simulink model "bb"  (R2014a)
settings: Solver=ode45  StartTime=0.0  StopTime=200  RelTol=1e-3
settings Model: Creator=York  LastModifiedBy=York

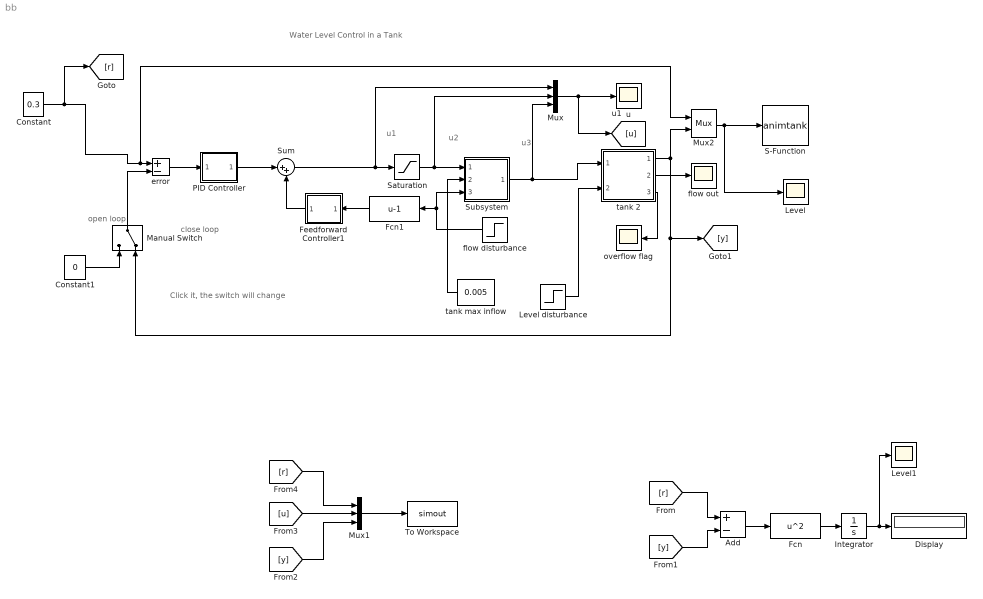
== system bb ==
  note: Water Level Control in a Tank
  note: open loop
  note: close loop
  note: Click it, the switch will change
  note: u1
  note: u2
  note: u3
  Add : Sum  Inputs=+-
  Constant : Constant  Value=0.3
  Constant1 : Constant  Value=0
  Display : Display
  Fcn : Fcn  Expr=u^2
  Fcn1 : Fcn  Expr=u-1
  Feedforward Controller1 : Subsystem  mask(feedforward Controller){K=0.002, T1=10, T2=2, t=8}
      mask prompts: K "Kffl:"; T1 "Tlead:"; T2 "Tlag:"; t "tff:"
      mask Display: disp('Gff(s)')
  Integrator : Integrator
  Level : Scope
      settings: TickLabels=on  TimeRange=200  YMin=-2.000000  YMax=2.000000  SaveName=ScopeData3
  Level disturbance : Step  Time=100  Before=1  SampleTime=0
  Level1 : Scope
      settings: TickLabels=on  TimeRange=200  YMin=-0.03  YMax=0  SaveName=ScopeData2
  Manual Switch : ManualSwitch  CurrentSetting=0
  Mux : Mux  Inputs=3
  Mux1 : Mux  Inputs=3
  Mux2 : Mux  Inputs=2
  PID Controller : Subsystem  mask(PID Controller){P=100, I=5, D=10}
      mask prompts: P "Proportional:"; I "Integral"; D "Derivative:"
      mask help:
      | Enter expressions for proportional, integral, and derivative terms.
      | P+I/s+Ds
      mask Help: This block implements a PID controller where parameters are entered for the Proportional, Integral and Derivative terms. Unmask this block to see how it works. The derivative term is implemented using a true derivative block.
      mask Display: disp('PID')
  S-Function : S-Function  FunctionName=animtank  Parameters=1  EnableBusSupport=off
  Saturation : Saturate  UpperLimit=1  LowerLimit=0
  Subsystem : Subsystem  mask(Valve){InitialPosition=1}
      mask prompts: InitialPosition "Initial position [0=closed 1=open]:"
      mask help: Valve
      mask Display: disp('VALVE')
  Sum : Sum  Inputs=|++
  To Workspace : ToWorkspace  VariableName=simout  SaveFormat=Structure With Time  SampleTime=-1
  error : Sum  Inputs=+-  SaturateOnIntegerOverflow=on  InputSameDT=on  OutDataTypeStr=Inherit: Same as first input
  flow disturbance : Step  Time=50  Before=1  SampleTime=0
  flow out : Scope
      settings: TickLabels=on  TimeRange=200.000000  YMin=-2.000000  YMax=2.000000  SaveName=ScopeData4
  overflow flag : Scope
      settings: TickLabels=on  TimeRange=20.000000  YMin=-2.000000  YMax=2.000000
  tank 2 : Subsystem  mask(Water tank){ht=0.45, area=0.12, outletArea=0.0008, overflowLimit=0, initialHt=0}
      mask prompts: ht "Height of tank (m):"; area "Bottom area (m^2):"; outletArea "Out pipe crossection (m^2):"; overflowLimit "Overflow sensor distance from top (m):"; initialHt "Initial level height (m):"
      mask help: Cylindrical water tank with overflow signal
      mask Display: disp('WATER\nTANK')
  tank max inflow : Constant  Value=0.005
  u : Scope
      settings: TickLabels=on  TimeRange=20  YMin=-2.000000  YMax=2.000000
  wires:
  tank 2/2(flow out) -> flow out/1
  tank max inflow/1 -> Subsystem/2(source flow)
  Subsystem/1(out flow) -> Mux/3, tank 2/1(flow in)
  tank 2/1(water level) -> Mux2/2, [y], Manual Switch/2
  tank 2/3(overflow flag) -> overflow flag/1
  Mux2/1 -> S-Function/1, Level/1
  Manual Switch/1 -> error/2
  Constant1/1 -> Manual Switch/1
  Constant/1 -> error/1, Mux2/1, [r]
  flow disturbance/1 -> Fcn1/1, Subsystem/3(flow disturbance)
  Level disturbance/1 -> tank 2/2(Level disturbance)
  Saturation/1 -> Mux/2, Subsystem/1(control)
  [r] -> Add/1
  [y] -> Add/2
  Add/1 -> Fcn/1
  Fcn/1 -> Integrator/1
  Integrator/1 -> Display/1, Level1/1
  Mux/1 -> u/1, [u]
  Mux1/1 -> To Workspace/1
  [r] -> Mux1/1
  [u] -> Mux1/2
  [y] -> Mux1/3
  Sum/1 -> Mux/1, Saturation/1
  Feedforward Controller1/1(Out_1) -> Sum/2
  error/1 -> PID Controller/1(In_1)
  PID Controller/1(Out_1) -> Sum/1
  Fcn1/1 -> Feedforward Controller1/1(In_1)

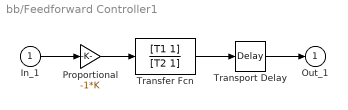
== system bb/Feedforward Controller1 ==
  In_1 : Inport
  Proportional : Gain  Gain=-1*K  SaturateOnIntegerOverflow=on  OutDataTypeStr=Inherit: Same as input  ParamDataTypeStr=Inherit: Same as input
  Transfer Fcn : TransferFcn  Numerator=[T1 1]  Denominator=[T2 1]
  Transport Delay : TransportDelay  DelayTime=t
  Out_1 : Outport  InitialOutput=0
  wires:
  In_1/1 -> Proportional/1
  Proportional/1 -> Transfer Fcn/1
  Transfer Fcn/1 -> Transport Delay/1
  Transport Delay/1 -> Out_1/1

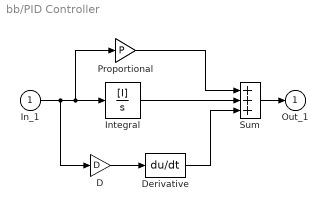
== system bb/PID Controller ==
  In_1 : Inport
  D : Gain  Gain=D  SaturateOnIntegerOverflow=on  OutDataTypeStr=Inherit: Same as input  ParamDataTypeStr=Inherit: Same as input
  Derivative : Derivative
  Integral : TransferFcn  Numerator=[I]  Denominator=[1 0]
  Proportional : Gain  Gain=P  SaturateOnIntegerOverflow=on  OutDataTypeStr=Inherit: Same as input  ParamDataTypeStr=Inherit: Same as input
  Sum : Sum  Inputs=+++  SaturateOnIntegerOverflow=on  InputSameDT=on  OutDataTypeStr=Inherit: Same as first input
  Out_1 : Outport  InitialOutput=0
  wires:
  Proportional/1 -> Sum/1
  Integral/1 -> Sum/2
  Derivative/1 -> Sum/3
  In_1/1 -> Integral/1, Proportional/1, D/1
  Sum/1 -> Out_1/1
  D/1 -> Derivative/1

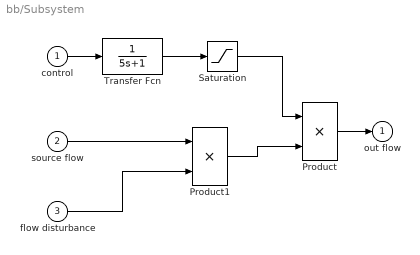
== system bb/Subsystem ==
  control : Inport
  source flow : Inport  Port=2
  flow disturbance : Inport  Port=3  OutMin=[0.1]  OutMax=[1.5]
  Product : Product  SaturateOnIntegerOverflow=on  RndMeth=Zero  InputSameDT=on  OutDataTypeStr=Inherit: Same as first input
  Product1 : Product  SaturateOnIntegerOverflow=on  RndMeth=Zero  InputSameDT=on  OutDataTypeStr=Inherit: Same as first input
  Saturation : Saturate  UpperLimit=1  LowerLimit=0
  Transfer Fcn : TransferFcn  Denominator=[5 1]
  out flow : Outport  InitialOutput=0
  wires:
  Product/1 -> out flow/1
  Saturation/1 -> Product/1
  Transfer Fcn/1 -> Saturation/1
  control/1 -> Transfer Fcn/1
  source flow/1 -> Product1/1
  Product1/1 -> Product/2
  flow disturbance/1 -> Product1/2

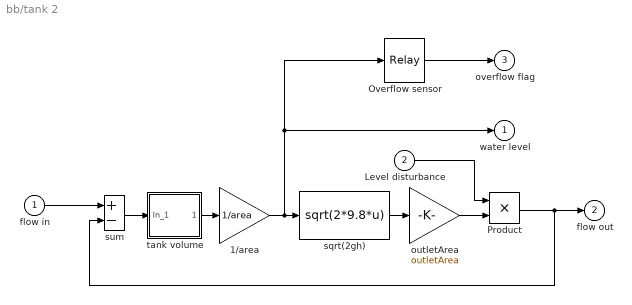
== system bb/tank 2 ==
  flow in : Inport
  Level disturbance : Inport  Port=2  OutMin=[0]  OutMax=[2]
  1/area : Gain  Gain=1/area  SaturateOnIntegerOverflow=on  OutDataTypeStr=Inherit: Same as input  ParamDataTypeStr=Inherit: Same as input
  Overflow sensor : Relay  OnSwitchValue=ht - overflowLimit  OffSwitchValue=ht - overflowLimit
  Product : Product  RndMeth=Zero
  outletArea : Gain  Gain=outletArea  SaturateOnIntegerOverflow=on  OutDataTypeStr=Inherit: Same as input  ParamDataTypeStr=Inherit: Same as input
  sqrt(2gh) : Fcn  Expr=sqrt(2*9.8*u)
  sum : Sum  Inputs=+-  SaturateOnIntegerOverflow=on  InputSameDT=on  OutDataTypeStr=Inherit: Same as first input
  tank volume : Subsystem  mask(Limited integrator.){lb=0, ub=ht * area, xi=initialHt * area}
      mask prompts: lb "Lower bound:"; ub "Upper bound:"; xi "Initial condition"
      mask help: Limited integrator
      mask Help: Implements a limited integrator with \nan expression of the form:\n\nif(x<=lb and u<0) or (x>=ub and u>0)\n\txdot=0\nelse\n\txdot=u.
      mask Display: plot(-1,-0.2,3.5,1.2,[0.05,1,2,2.9],[0,0,1,1]);disp(' 1/s    ')
  water level : Outport  InitialOutput=0
  flow out : Outport  Port=2  InitialOutput=0
  overflow flag : Outport  Port=3  InitialOutput=0
  wires:
  sqrt(2gh)/1 -> outletArea/1
  1/area/1 -> Overflow sensor/1, water level/1, sqrt(2gh)/1
  tank volume/1(Out_1) -> 1/area/1
  Overflow sensor/1 -> overflow flag/1
  flow in/1 -> sum/1
  sum/1 -> tank volume/1(In_1)
  outletArea/1 -> Product/2
  Product/1 -> flow out/1, sum/2
  Level disturbance/1 -> Product/1

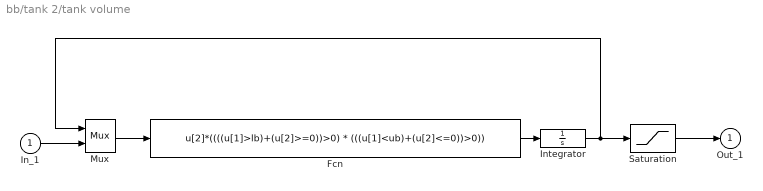
== system bb/tank 2/tank volume ==
  In_1 : Inport
  Fcn : Fcn  Expr=u[2]*((((u[1]>lb)+(u[2]>=0))>0) * (((u[1]<ub)+(u[2]<=0))>0))
  Integrator : Integrator  InitialCondition=xi
  Mux : Mux  Inputs=2
  Saturation : Saturate  UpperLimit=ub  LowerLimit=lb
  Out_1 : Outport  InitialOutput=0
  wires:
  Integrator/1 -> Saturation/1, Mux/1
  Fcn/1 -> Integrator/1
  Mux/1 -> Fcn/1
  In_1/1 -> Mux/2
  Saturation/1 -> Out_1/1
